simulink model "manual"  (R2021b)
settings: Solver=ode4  StartTime=0.0  StopTime=3000  FixedStep=1  RelTol=1e-3
libraries: simulink_extras x2
settings Model: Creator=shao  LastModifiedBy=shao
settings SolverCC: AlgebraicLoopSolver=TrustRegion
settings DebuggingCC: SFMachineParentedDataDiag=warning

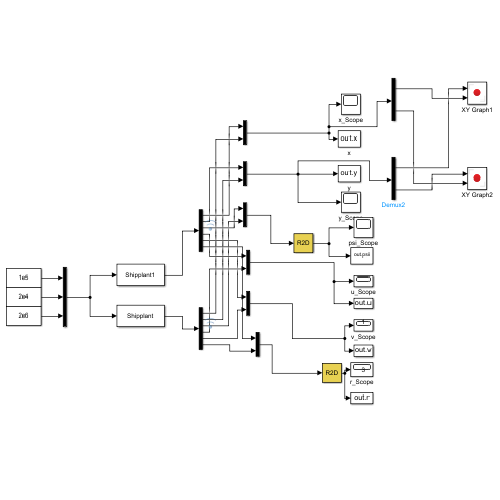
[thumbnail: Simulink's stored preview of the top-level diagram]
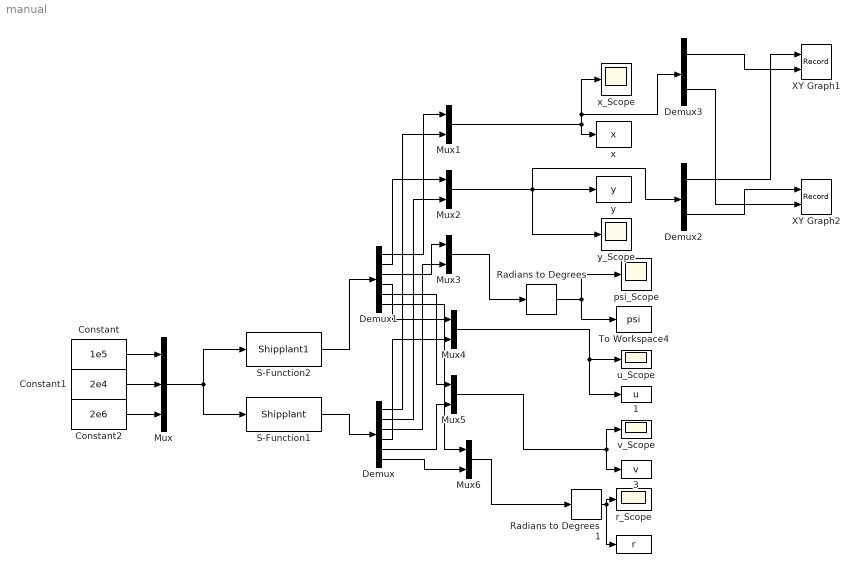
== system manual ==
  " " : ToWorkspace  VariableName=r  SampleTime=-1
  " 1" : ToWorkspace  VariableName=u  SampleTime=-1
  " 3" : ToWorkspace  VariableName=v  SampleTime=-1
  Constant : Constant  Value=1e5
  Constant1 : Constant  Value=2e4
  Constant2 : Constant  Value=2e6
  Demux : Demux  Outputs=6
      settings: DisplayOption=none
  Demux1 : Demux  Outputs=6
      settings: DisplayOption=none
  Demux2 : Demux  Outputs=2
      settings: DisplayOption=none
  Demux3 : Demux  Outputs=2
      settings: DisplayOption=none
  Mux : Mux  Inputs=3
  Mux{1..6} (6 alike) : Mux  Inputs=2
  "Radians to Degrees  " : simulink_extras/Transformations/Radians to Degrees
  Radians to Degrees  1 : simulink_extras/Transformations/Radians to Degrees
  S-Function1 : S-Function  FunctionName=Shipplant  SFunctionDeploymentMode=off  EnableBusSupport=off
  S-Function2 : S-Function  FunctionName=Shipplant1  SFunctionDeploymentMode=off  EnableBusSupport=off
  To Workspace4 : ToWorkspace  VariableName=psi  SampleTime=-1
  XY Graph1 : Record  FileSettingsInternal="{\"entries\":[{\"content\":{\"excelSettings\":{\"content\":{},\"type\":\"Streamout.ExcelSettings\"}},\"type\":\"Streamout.FileSettingStorage\",\"uuid\":\"8d99c108-ed2b-43d3-944a-b6be10a43ccc\"}],\"packageUris\":[\"http://schema.mathworks.com/mf0/streamout_blocks/R2020a\"],\"version\":\"1.0\"}"  Layout=[1 1]  SignalsInternal="{\"entries\":[{\"content\":{\"signals\":[{\"content\":{\"blockPath\":[\"manual/XY Graph1\"],\"channel\":[],\"dimensions\":[1],\"domain\":\"manual/XY Graph1\",\"lineColor\":\"#a2142f\",\"plots\":[1],\"port\":1,\"sid\":[\"\"],\"signalID\":2737,\"signalName\":\"Demux2:1\"},\"type\":\"RecordBlkView.Signal\",\"uuid\":\"b74782f7-3a1e-4437-a865-7b3f49e0818d\"},{\"content\":{\"blockPath\":[\"manual/XY Graph1\"],\"channel\":[],\"dimensions\":[1],\"domain\":\"manual/XY Graph1\",\"lineColor\":\"#139fff\",\"plots\":[1],\"port\":2,\"sid\":[\"\"],\"signalID\":2741,\"signalName\":\"Demux3:1\"},\"type\":\"RecordBlkView.Signal\",\"uuid\":\"2a70fe65-4d90-447b-9181-ebe2d87390e3\"}]},\"type\":\"RecordBlkView.InputSignals\",\"uuid\":\"b5d78593-1baa-4b93-a902-4e67342afc91\"}],\"packageUris\":[\"http://schema.mathworks.com/mf0/streamout_blocks/R2020a\"],\"version\":\"1.0\"}"  VisualizationBindings="{\"xyplotplugin\":{\"info\":[{\"series\":[{\"bindingParametersList\":[{\"parameter\":\"Y-Axis\",\"signalID\":2741,\"signalName\":\"Demux3:1\"},{\"parameter\":\"X-Axis\",\"signalID\":2737,\"signalName\":\"Demux2:1\"}],\"seriesID\":23456}],\"subplotID\":1}]}}"  CompatibilityTag=XY  st=-1
  XY Graph2 : Record  FileSettingsInternal="{\"entries\":[{\"content\":{\"excelSettings\":{\"content\":{},\"type\":\"Streamout.ExcelSettings\"}},\"type\":\"Streamout.FileSettingStorage\",\"uuid\":\"f1b0bad3-2038-40a4-a1d7-b18e059aa188\"}],\"packageUris\":[\"http://schema.mathworks.com/mf0/streamout_blocks/R2020a\"],\"version\":\"1.0\"}"  Layout=[1 1]  SignalsInternal="{\"entries\":[{\"content\":{\"signals\":[{\"content\":{\"blockPath\":[\"manual/XY Graph2\"],\"channel\":[],\"dimensions\":[1],\"domain\":\"manual/XY Graph2\",\"lineColor\":\"#a2142f\",\"plots\":[1],\"port\":1,\"sid\":[],\"signalID\":3254,\"signalName\":\"x\"},\"type\":\"RecordBlkView.Signal\",\"uuid\":\"72da7f81-ea3d-4916-857f-73d7643b0373\"},{\"content\":{\"blockPath\":[\"manual/XY Graph2\"],\"channel\":[],\"dimensions\":[1],\"domain\":\"manual/XY Graph2\",\"lineColor\":\"#139fff\",\"plots\":[1],\"port\":2,\"sid\":[],\"signalID\":3257,\"signalName\":\"y\"},\"type\":\"RecordBlkView.Signal\",\"uuid\":\"de010768-395a-458f-ac7e-0eadac0fcedf\"}]},\"type\":\"RecordBlkView.InputSignals\",\"uuid\":\"383b3363-b0e8-4e2b-9d60-651d58551ca8\"}],\"packageUris\":[\"http://schema.mathworks.com/mf0/streamout_blocks/R2020a\"],\"version\":\"1.0\"}"  VisualizationBindings="{\"xyplotplugin\":{\"info\":[{\"series\":[{\"bindingParametersList\":[{\"parameter\":\"Y-Axis\",\"signalID\":3257,\"signalName\":\"y\"},{\"parameter\":\"X-Axis\",\"signalID\":3254,\"signalName\":\"x\"}],\"seriesID\":32245}],\"subplotID\":1}]}}"  CompatibilityTag=XY  st=-1
  psi_Scope : Scope
  r_Scope : Scope
  u_Scope : Scope
  v_Scope : Scope
  x : ToWorkspace  VariableName=x  SampleTime=-1
  x_Scope : Scope
  y : ToWorkspace  VariableName=y  SampleTime=-1
  y_Scope : Scope
  wires:
  Mux/1 -> S-Function2/1, S-Function1/1
  Constant/1 -> Mux/1
  Constant1/1 -> Mux/2
  Constant2/1 -> Mux/3
  Mux1/1 -> Demux3/1, x_Scope/1, x/1
  Mux2/1 -> y_Scope/1, y/1, Demux2/1
  Mux5/1 -> v_Scope/1, " 3"/1
  Mux4/1 -> " 1"/1, u_Scope/1
  Radians to Degrees  1/1 -> " "/1, r_Scope/1
  "Radians to Degrees  "/1 -> To Workspace4/1, psi_Scope/1
  Mux3/1 -> "Radians to Degrees  "/1
  Mux6/1 -> Radians to Degrees  1/1
  S-Function2/1 -> Demux1/1
  S-Function1/1 -> Demux/1
  Demux1/1 -> Mux1/1
  Demux/1 -> Mux1/2
  Demux1/2 -> Mux2/1
  Demux/2 -> Mux2/2
  Demux1/3 -> Mux3/1
  Demux/3 -> Mux3/2
  Demux1/4 -> Mux4/1
  Demux/4 -> Mux4/2
  Demux1/5 -> Mux5/1
  Demux/5 -> Mux5/2
  Demux/6 -> Mux6/2
  Demux1/6 -> Mux6/1
  Demux3/1 -> XY Graph1/2
  Demux2/1 -> XY Graph1/1
  Demux3/2 -> XY Graph2/2
  Demux2/2 -> XY Graph2/1
